simulink model "SigProcessFinished"  (R2022b)
settings: configuration reference "TmVcThermal_Configuration_sub" (kept outside this file)
undefined symbols (not defined in the file): cClCddAdc_D_u16ADNum, cClCddAdc_D_u8FilterType, cClCddAdc_D_u8RawValueNum
libraries: simulink x23
(part 2 of 2)

== matlab function SigProcessFinished/SigProcessSub/CLHB02001_Filter/AVG5/MATLAB Function ==
  data: u input; mid output; withoutEdge output; num input

function [mid, withoutEdge] = fcn(u,num)
% 输入u: 待排序数组
% 输入num: 滤波个数，max is 20
n = num;
for i = 1:n-1
    for j = 1:n-i
        if u(j) > u(j+1)
            temp = u(j);
            u(j) = u(j+1);
            u(j+1) = temp;
        end
    end
end
sortedData = u;

mid = sortedData(ceil(num/2)); % 取中间值
withoutEdge = mean(sortedData(2:num-1));

== matlab function SigProcessFinished/SigProcessSub/CLHB02001_Filter/AVG6/MATLAB Function ==
  data: u input; mid output; withoutEdge output; num input

function [mid, withoutEdge] = fcn(u,num)
% 输入u: 待排序数组
% 输入num: 滤波个数，max is 20
n = num;
for i = 1:n-1
    for j = 1:n-i
        if u(j) > u(j+1)
            temp = u(j);
            u(j) = u(j+1);
            u(j+1) = temp;
        end
    end
end
sortedData = u;

mid = sortedData(ceil(num/2)); % 取中间值
withoutEdge = mean(sortedData(2:num-1));

== matlab function SigProcessFinished/SigProcessSub/CLHB02001_Filter/AVG7/MATLAB Function ==
  data: u input; mid output; withoutEdge output; num input

function [mid, withoutEdge] = fcn(u,num)
% 输入u: 待排序数组
% 输入num: 滤波个数，max is 20
n = num;
for i = 1:n-1
    for j = 1:n-i
        if u(j) > u(j+1)
            temp = u(j);
            u(j) = u(j+1);
            u(j+1) = temp;
        end
    end
end
sortedData = u;

mid = sortedData(ceil(num/2)); % 取中间值
withoutEdge = mean(sortedData(2:num-1));

== matlab function SigProcessFinished/SigProcessSub/CLHB02001_Filter/AVG8/MATLAB Function ==
  data: u input; mid output; withoutEdge output; num input

function [mid, withoutEdge] = fcn(u,num)
% 输入u: 待排序数组
% 输入num: 滤波个数，max is 20
n = num;
for i = 1:n-1
    for j = 1:n-i
        if u(j) > u(j+1)
            temp = u(j);
            u(j) = u(j+1);
            u(j+1) = temp;
        end
    end
end
sortedData = u;

mid = sortedData(ceil(num/2)); % 取中间值
withoutEdge = mean(sortedData(2:num-1));

== matlab function SigProcessFinished/SigProcessSub/CLHB02001_Filter/AVG9/MATLAB Function ==
  data: u input; mid output; withoutEdge output; num input

function [mid, withoutEdge] = fcn(u,num)
% 输入u: 待排序数组
% 输入num: 滤波个数，max is 20
n = num;
for i = 1:n-1
    for j = 1:n-i
        if u(j) > u(j+1)
            temp = u(j);
            u(j) = u(j+1);
            u(j+1) = temp;
        end
    end
end
sortedData = u;

mid = sortedData(ceil(num/2)); % 取中间值
withoutEdge = mean(sortedData(2:num-1));
